simulink model "BaseEngineController_LS"  (Simulink 7.7)
settings: Solver=FixedStepDiscrete  StartTime=0.0  StopTime=10.0  RelTol=1e-3
PreLoadFcn:
  | try, eval([bdroot '_setup']); catch, eval('model_setup', ''); end
InitFcn:
  | try, eval([bdroot '_setup']); catch, eval('model_setup', ''); end
undefined symbols (not defined in the file): ECU555, High, motohawk_build_version, motohawk_trunc_name, motohawk_vardec_config_group, motohawk_vardec_path, True
libraries: MotoHawk_lib x1418, motohawk_control_primitives_lib x183, motohawk_engine_lib x32, simulink x21, motohawk_annotations_lib x9, AutoDoc_lib x8, simulink_extras x4, motohawk_ccp_examples_lib x1, motohawk_control_primitives_motoshare_lib x1
(part 3 of 27)

== system BaseEngineController_LS/Foreground/Inputs/PotentiometerSensors ==
  APP1 : Subsystem  AncestorBlock=motohawk_engine_lib/Non-Linear Sensor Characterization (tbl)  mask(Non-Linear Sensor Characterization (tbl)){nam='APP1', prefix='APP1', units='%', inputunits='ADC', parent_group=motohawk_vardec_path(gcb), tblsize=9, samp_time=-1}
      mask prompts: nam "Name"; units "Output Units"; inputunits "Input Units"; parent_group "MotoTune Group"; tblsize "Table Size"; samp_time "Sample Time"
      mask help:
      | Converts from A/D Counts to Engineering Units using a 1-D Table Lookup.
      | Saturates the converted value around Min and Max values and triggers a Fault when out of range.
      mask init:
      | lbl = ['Non-Linear Sensor (tbl): ' nam ' [' units ']'];
      | group = [parent_group ' | ' nam];
      settings: RTWSystemCode=Function  RTWFcnNameOpts=Use subsystem name  RTWFileNameOpts=Use function name
      mask Display:
      | patch([0 0 1 1], [0 0.075 0.075 0], [230/255 0/255 0/255])
      | patch([0 0 1 1], [0.025 0.05 0.05 0.025], [150/255 0/255 0/255])
      | patch([0 0 1 1], [0 0.025 0.025 0], [0/255 0/255 0/255])
      | 
      | disp(lbl);
  APP1ForcedAdapt : Subsystem
  APP2 : Subsystem  AncestorBlock=motohawk_engine_lib/Non-Linear Sensor Characterization (tbl)  mask(Non-Linear Sensor Characterization (tbl)){nam='APP2', prefix='APP2', units='%', inputunits='ADC', parent_group=motohawk_vardec_path(gcb), tblsize=9, samp_time=-1}
      mask prompts: nam "Name"; units "Output Units"; inputunits "Input Units"; parent_group "MotoTune Group"; tblsize "Table Size"; samp_time "Sample Time"
      mask help:
      | Converts from A/D Counts to Engineering Units using a 1-D Table Lookup.
      | Saturates the converted value around Min and Max values and triggers a Fault when out of range.
      mask init:
      | lbl = ['Non-Linear Sensor (tbl): ' nam ' [' units ']'];
      | group = [parent_group ' | ' nam];
      settings: RTWSystemCode=Function  RTWFcnNameOpts=Use subsystem name  RTWFileNameOpts=Use function name
      mask Display:
      | patch([0 0 1 1], [0 0.075 0.075 0], [230/255 0/255 0/255])
      | patch([0 0 1 1], [0.025 0.05 0.05 0.025], [150/255 0/255 0/255])
      | patch([0 0 1 1], [0 0.025 0.025 0], [0/255 0/255 0/255])
      | 
      | disp(lbl);
  APP2ForcedAdapt : Subsystem
  Bus Creator1 : BusCreator
  Constant4 : Constant  Value=false
  Constant5 : Constant  Value=false
  Linear Sensor Characterization w Adapt : motohawk_engine_lib/Linear Sensor Characterization w Adapt  SystemSampleTime=-1  nam='APP1_Adapt'  prefix='APP1_Adapt'  samp_time=-1  parent_group=motohawk_vardec_path(gcb)
  Linear Sensor Characterization w Adapt1 : motohawk_engine_lib/Linear Sensor Characterization w Adapt  SystemSampleTime=-1  nam='APP2_Adapt'  prefix='APP2_Adapt'  samp_time=-1  parent_group=motohawk_vardec_path(gcb)
  Switch : Switch  Criteria=u2 ~= 0
  Switch1 : Switch  Criteria=u2 ~= 0
  TPS1 : motohawk_engine_lib/Linear Sensor Characterization w Adapt  SystemSampleTime=-1  nam='TPS1'  prefix='TPS1'  samp_time=-1  parent_group=motohawk_vardec_path(gcb)
  TPS2 : motohawk_engine_lib/Linear Sensor Characterization w Adapt  SystemSampleTime=-1  nam='TPS2'  prefix='TPS2'  samp_time=-1  parent_group=motohawk_vardec_path(gcb)
  Terminator{2..5,10..11} (6 alike) : Terminator
  motohawk_ain1 : MotoHawk_lib/Analog I//O Blocks/motohawk_ain  res_name=[]  text_resource=AN5M  code_resource=RES_ECUP  val_resource=-1  target=ECU555-80  resource_enum_str=(None)=-1,ECUP=53,DRVP=54,XDRP=55,AN1M=56,AN2M=57,AN3M=58,AN4M=59,AN5M=60,AN6M=61,AN7M=62,AN8M=63,AN9M=64,AN10M=65,AN11M=66,AN12M=67,AN13M=68,AN14M=69,AN15M=70,AN16M=71,AN17M=72,AN18M=73,AN19M=74,O2A=90,O2B=91,XDRP_B=92  altref=5V Reference  typ=uint16  num_adc_bits=10  use_stat=off  use_vardec=on  nam='APP1AnalogInput'  read_level=1  write_level=1  group='System | I/O Pins | Inputs Config'
  motohawk_ain2 : MotoHawk_lib/Analog I//O Blocks/motohawk_ain  res_name=[]  text_resource=AN4M  code_resource=RES_ECUP  val_resource=-1  target=ECU555-80  resource_enum_str=(None)=-1,ECUP=53,DRVP=54,XDRP=55,AN1M=56,AN2M=57,AN3M=58,AN4M=59,AN5M=60,AN6M=61,AN7M=62,AN8M=63,AN9M=64,AN10M=65,AN11M=66,AN12M=67,AN13M=68,AN14M=69,AN15M=70,AN16M=71,AN17M=72,AN18M=73,AN19M=74,O2A=90,O2B=91,XDRP_B=92  altref=5V Reference  typ=uint16  num_adc_bits=10  use_stat=off  use_vardec=on  nam='APP2AnalogInput'  read_level=1  write_level=1  group='System | I/O Pins | Inputs Config'
  motohawk_ain6 : MotoHawk_lib/Analog I//O Blocks/motohawk_ain  res_name=[]  text_resource=AN5M  code_resource=RES_ECUP  val_resource=-1  target=ECU555-80  resource_enum_str=(None)=-1,ECUP=53,DRVP=54,XDRP=55,AN1M=56,AN2M=57,AN3M=58,AN4M=59,AN5M=60,AN6M=61,AN7M=62,AN8M=63,AN9M=64,AN10M=65,AN11M=66,AN12M=67,AN13M=68,AN14M=69,AN15M=70,AN16M=71,AN17M=72,AN18M=73,AN19M=74,O2A=90,O2B=91,XDRP_B=92  altref=5V Reference  typ=uint16  num_adc_bits=10  use_stat=off  use_vardec=on  nam='TPS1AnalogInput'  read_level=1  write_level=1  group='System | I/O Pins | Inputs Config'
  motohawk_ain9 : MotoHawk_lib/Analog I//O Blocks/motohawk_ain  res_name=[]  text_resource=AN4M  code_resource=RES_ECUP  val_resource=-1  target=ECU555-80  resource_enum_str=(None)=-1,ECUP=53,DRVP=54,XDRP=55,AN1M=56,AN2M=57,AN3M=58,AN4M=59,AN5M=60,AN6M=61,AN7M=62,AN8M=63,AN9M=64,AN10M=65,AN11M=66,AN12M=67,AN13M=68,AN14M=69,AN15M=70,AN16M=71,AN17M=72,AN18M=73,AN19M=74,O2A=90,O2B=91,XDRP_B=92  altref=5V Reference  typ=uint16  num_adc_bits=10  use_stat=off  use_vardec=on  nam='TPS2AnalogInput'  read_level=1  write_level=1  group='System | I/O Pins | Inputs Config'
  motohawk_calibration : MotoHawk_lib/Calibration & Probing Blocks/motohawk_calibration  nam='APP_AdaptMode'  val=0  storage=Calibration  show_more=on  name_source=Use Parameter  data_type=boolean  read_level=1  write_level=1  ovr_cals=on  view_as=Enumeration  enum_struct={'Disabled', 'Enabled'}  vector_style=Wide Row  use_help_units=off  help=''  units=''  use_header_enum=off  row_header_enum={}  col_header_enum={}  use_min_max=off  min_val=-inf  max_val=inf  use_precision=off  precision=''  gain=1  offset=0  exp=1  use_mototune_group=on  mototune_group=motohawk_vardec_path(gcb)
  motohawk_callout1 : motohawk_annotations_lib/motohawk_callout1  BlockType_='Mototron_harea'  desc='\fontsize{12}Read from H/W'  edit_text=Compute the mean forward body acceleration.Worry about rounding.  edit_as=255
  motohawk_callout2 : motohawk_annotations_lib/motohawk_callout1  BlockType_='Mototron_harea'  desc='\fontsize{12}Convert to Engineering Units'  edit_text=Compute the mean forward body acceleration.Worry about rounding.  edit_as=255
  motohawk_callout3 : motohawk_annotations_lib/motohawk_callout1  BlockType_='Mototron_harea'  desc='\fontsize{12}Create a Bus of Sensors'  edit_text=Compute the mean forward body acceleration.Worry about rounding.  edit_as=255
  motohawk_data_read : MotoHawk_lib/Data Storage Blocks/motohawk_data_read  source=Lookup By Name  structure=Scalar  operation=Read scalar from location by index  sz_vec=4  sz_row=2  sz_col=3  typ=boolean  nam='TPSAdaptLoRequest'  checkNull=on  struct_inst_name='Struct1'  struct_nam='MyStruct'
  SensorBus : Outport
  wires:
  Bus Creator1/1 -> SensorBus/1  "PotSensors"
  motohawk_ain1/1 -> APP1/1(ADC), Linear Sensor Characterization w Adapt/1
  motohawk_ain2/1 -> APP2/1(ADC), Linear Sensor Characterization w Adapt1/1
  APP1/2(EngUnitsRaw) -> Terminator2/1
  APP2/2(EngUnitsRaw) -> Terminator3/1
  Linear Sensor Characterization w Adapt/2 -> Terminator4/1
  APP1ForcedAdapt/1(LowSide Request) -> Linear Sensor Characterization w Adapt/2
  APP1ForcedAdapt/2(HiSide Request) -> Linear Sensor Characterization w Adapt/3
  APP2ForcedAdapt/1(LowSide Request) -> Linear Sensor Characterization w Adapt1/2
  APP2ForcedAdapt/2(HiSide Request) -> Linear Sensor Characterization w Adapt1/3
  Linear Sensor Characterization w Adapt1/2 -> Terminator5/1
  Constant4/1 -> TPS1/3
  motohawk_data_read/1 -> TPS2/2, TPS1/2
  TPS2/2 -> Terminator11/1
  TPS1/2 -> Terminator10/1
  motohawk_ain6/1 -> TPS1/1
  motohawk_ain9/1 -> TPS2/1
  APP1/1(EngUnitsFilt) -> Switch/3  "APP1"
  Linear Sensor Characterization w Adapt/1 -> Switch/1
  APP2/1(EngUnitsFilt) -> Switch1/3  "APP2"
  Linear Sensor Characterization w Adapt1/1 -> Switch1/1
  motohawk_calibration/1 -> Switch/2, Switch1/2
  Switch/1 -> Bus Creator1/1  "APP1"
  Switch1/1 -> Bus Creator1/2  "APP2"
  TPS1/1 -> Bus Creator1/3  "TPS1"
  TPS2/1 -> Bus Creator1/4  "TPS2"
  Constant5/1 -> TPS2/3

== system BaseEngineController_LS/Foreground/Outputs/AC Control ==
  AC : Inport
  Discrete Actuator - AC : motohawk_engine_lib/Discrete Actuator Characterization  SystemSampleTime=-1  prefix='AC'  nam='AC'  units='bool'  parent_group=motohawk_vardec_path(gcb)  polarity=High-True
  motohawk_dout : MotoHawk_lib/Digital I//O Blocks/motohawk_dout  resource_name=[]  text_resource=(None)  target=ECU555-80  use_diag=off  use_vardec=on  nam='ACPin'  read_level=1  write_level=1  group='System | I/O Pins | Outputs Config'
  wires:
  Discrete Actuator - AC/1 -> motohawk_dout/1
  AC/1 -> Discrete Actuator - AC/1

== system BaseEngineController_LS/Foreground/Outputs/AEM Infinity Dash ==
  Data : Inport
  Dash Custom 1 : Subsystem
  Dash Message 1 : Subsystem
  Dash Message 2 : Subsystem
  Dash Message 3 : Subsystem
  Dash Message 4 : Subsystem
  Dash Message 5 : Subsystem
  Dash Message 6 : Subsystem
  Dash Message 7 : Subsystem
  Dash Message 8 : Subsystem
  Dash Message Boost : Subsystem
  Dash Message DBW : Subsystem
  wires:
  Data/1 -> Dash Message 1/1(Data), Dash Message 2/1(Data), Dash Message 3/1(Data), Dash Message 4/1(Data), Dash Message 6/1(Data), Dash Message Boost/1(Data), Dash Message DBW/1(Data), Dash Custom 1/1(Data), Dash Message 5/1(Data)

== system BaseEngineController_LS/Foreground/Outputs/Coil Control ==
  SparkEnable : Inport
  SparkStartAngle : Inport  Port=2
  SparkAdvance : Inport  Port=3
  CutSequence : Inport  Port=4
  Trigger : TriggerPort  TriggerType=function-call
  Coil Enable Manager : Subsystem
  Data Type Conversion : DataTypeConversion  SaturateOnIntegerOverflow=on  RndMeth=Zero
  Data Type Conversion1 : DataTypeConversion  SaturateOnIntegerOverflow=on  RndMeth=Zero
  Data Type Conversion2 : DataTypeConversion  SaturateOnIntegerOverflow=on  RndMeth=Zero
  EST Fault Management : Subsystem
  Gain : Gain  Gain=16  SaturateOnIntegerOverflow=on  OutDataTypeStr=Inherit: Same as input  ParamDataTypeStr=Inherit: Same as input
  Gain1 : Gain  Gain=16  SaturateOnIntegerOverflow=on  OutDataTypeStr=Inherit: Same as input  ParamDataTypeStr=Inherit: Same as input
  Gain2 : Gain  Gain=1000  SaturateOnIntegerOverflow=on  OutDataTypeStr=Inherit: Same as input  ParamDataTypeStr=Inherit: Same as input
  Logical Operator1 : Logic  Inputs=3  AllPortsSameDT=off  OutDataTypeStr=boolean
  Spark Sequence : MotoHawk_lib/Advanced Digital I//O/Spark Sequence  text_resource=EST 1  code_resource=RES_EST1  val_resource=-1  target=ECU555-80  resource_enum_str=(None)=-1,EST 1=36,EST 2=37,EST 3=38,EST 4=39,EST 5=40,EST 6=41,EST 7=42,EST 8=43  sequence_type=Standard (Coil per cylinder)  stop_mode=Angle Controlled  update_mode=OS  granularity=Fine  min_duration_mode=Static  min_duration=1.5  use_diag=on  open_threshold=500  use_vardec=on  nam='EST_'  read_level=1  write_level=1  group='System | I/O Pins | Outputs Config'
  motohawk_calibration2 : MotoHawk_lib/Calibration & Probing Blocks/motohawk_calibration  nam='SparkMaxDuration'  val=5  storage=Calibration  show_more=on  name_source=Use Parameter  data_type=Inherit via back propagation  read_level=1  write_level=1  ovr_cals=on  view_as=Number  enum_struct={'Disabled', 'Enabled'}  vector_style=Wide Row  use_help_units=on  help="'Maximum duration for a spark pulse.  Must be a multiple of 5ms'"  units='ms'  use_header_enum=off  row_header_enum={}  col_header_enum={}  use_min_max=off  min_val=-inf  max_val=inf  use_precision=off  precision=''  gain=1  offset=0  exp=1  use_mototune_group=on  mototune_group=motohawk_vardec_path(gcb)
  motohawk_override_rel : MotoHawk_lib/Calibration & Probing Blocks/motohawk_override_rel  SystemSampleTime=-1  parent_name='SparkStartAngle'  show_more=on  name_source=Use Parameter  parent_read_level=1  parent_override_level=1  use_help_units=on  parent_help='Provides a relative offset to input signal'  parent_units='degBTDC'  use_min_max=off  parent_min=-inf  parent_max=inf  use_precision=off  parent_precision=''  parent_gain=1  parent_offset=0  parent_exp=1  use_mototune_group=on  parent_group=motohawk_vardec_path(gcb)
  motohawk_override_rel1 : MotoHawk_lib/Calibration & Probing Blocks/motohawk_override_rel  SystemSampleTime=-1  parent_name='SparkStopAngle'  show_more=on  name_source=Use Parameter  parent_read_level=1  parent_override_level=1  use_help_units=on  parent_help='Provides a relative offset to input signal'  parent_units='degBTDC'  use_min_max=off  parent_min=-inf  parent_max=inf  use_precision=off  parent_precision=''  parent_gain=1  parent_offset=0  parent_exp=1  use_mototune_group=on  parent_group=motohawk_vardec_path(gcb)
  motohawk_probe : MotoHawk_lib/Calibration & Probing Blocks/motohawk_probe  nam='CoilStartAngle'  show_more=on  name_source=Use Parameter  read_level=1  view_as=Number  enum_struct={'Disabled', 'Enabled'}  vector_style=Wide Row  use_help_units=on  help='StartAngle for coils to establish dwell.'  units='degBTDC'  use_header_enum=off  row_header_enum={}  col_header_enum={}  use_precision=off  precision=''  gain=1  offset=0  exp=1  use_mototune_group=on  mototune_group=motohawk_vardec_path(gcb)
  motohawk_probe1 : MotoHawk_lib/Calibration & Probing Blocks/motohawk_probe  nam='CoilStopAngle'  show_more=on  name_source=Use Parameter  read_level=1  view_as=Number  enum_struct={'Disabled', 'Enabled'}  vector_style=Wide Row  use_help_units=on  help='Stop angle for coils to establish dwell.'  units='degBTDC'  use_header_enum=off  row_header_enum={}  col_header_enum={}  use_precision=off  precision=''  gain=1  offset=0  exp=1  use_mototune_group=on  mototune_group=motohawk_vardec_path(gcb)
  motohawk_probe2 : MotoHawk_lib/Calibration & Probing Blocks/motohawk_probe  nam='CoilEnabled'  show_more=on  name_source=Use Parameter  read_level=1  view_as=Number  enum_struct={'Disabled', 'Enabled'}  vector_style=Wide Row  use_help_units=on  help='Enable sate for coils.'  units='bool'  use_header_enum=off  row_header_enum={}  col_header_enum={}  use_precision=off  precision=''  gain=1  offset=0  exp=1  use_mototune_group=on  mototune_group=motohawk_vardec_path(gcb)
  wires:
  CutSequence/1 -> Logical Operator1/3
  SparkEnable/1 -> Logical Operator1/2
  Coil Enable Manager/1(Enable) -> Logical Operator1/1
  Gain2/1 -> Data Type Conversion2/1
  Data Type Conversion2/1 -> Spark Sequence/4
  motohawk_override_rel/1 -> motohawk_probe/1, Gain/1
  motohawk_override_rel1/1 -> motohawk_probe1/1, Gain1/1
  Logical Operator1/1 -> motohawk_probe2/1, Spark Sequence/1
  SparkAdvance/1 -> motohawk_override_rel1/1
  SparkStartAngle/1 -> motohawk_override_rel/1
  motohawk_calibration2/1 -> Gain2/1
  Data Type Conversion1/1 -> Spark Sequence/3
  Data Type Conversion/1 -> Spark Sequence/2
  Gain1/1 -> Data Type Conversion1/1
  Gain/1 -> Data Type Conversion/1
  Spark Sequence/1 -> EST Fault Management/1(Short)
  Spark Sequence/2 -> EST Fault Management/2(Open)
  Spark Sequence/3 -> EST Fault Management/3(OpenADC)
  Spark Sequence/4 -> EST Fault Management/4(Dwell)

== system BaseEngineController_LS/Foreground/Outputs/ETC_CutPower ==
  ETC : Inport
  ESTOP : Inport  Port=2
  TimeSinceStall : Inport  Port=3
  Logical Operator : Logic  AllPortsSameDT=off  OutDataTypeStr=boolean
  Logical Operator9 : Logic  Operator=OR  AllPortsSameDT=off  OutDataTypeStr=boolean
  Relational Operator : RelationalOperator  Operator=<  OutDataTypeStr=boolean
  Relational Operator3 : RelationalOperator  Operator=>  ZeroCross=off  InputSameDT=on
  motohawk_calibration1 : MotoHawk_lib/Calibration & Probing Blocks/motohawk_calibration  nam='ETC_CutPower_ETC'  val=20  storage=Calibration  show_more=on  name_source=Use Parameter  data_type=Inherit from 'Default Value'  read_level=1  write_level=1  ovr_cals=on  view_as=Number  enum_struct={'Disabled', 'Enabled'}  vector_style=Wide Row  use_help_units=on  help='Cut power to ETC if ETC request is less than this'  units='%'  use_header_enum=off  row_header_enum={}  col_header_enum={}  use_min_max=on  min_val=0  max_val=100  use_precision=on  precision='2.3'  gain=1  offset=0  exp=1  use_mototune_group=on  mototune_group=motohawk_vardec_path(gcb)
  motohawk_calibration3 : MotoHawk_lib/Calibration & Probing Blocks/motohawk_calibration  nam='ETC_CutPower_StallTime'  val=15  storage=Calibration  show_more=on  name_source=Use Parameter  data_type=Inherit from 'Default Value'  read_level=1  write_level=1  ovr_cals=on  view_as=Number  enum_struct={'Disabled', 'Enabled'}  vector_style=Wide Row  use_help_units=on  help='Cut power to ETC after stalled this long'  units='s'  use_header_enum=off  row_header_enum={}  col_header_enum={}  use_min_max=off  min_val=0  max_val=100  use_precision=on  precision='2.3'  gain=1  offset=0  exp=1  use_mototune_group=on  mototune_group=motohawk_vardec_path(gcb)
  ETC OFF : Outport
  wires:
  ESTOP/1 -> Logical Operator9/1
  TimeSinceStall/1 -> Relational Operator3/1
  motohawk_calibration3/1 -> Relational Operator3/2
  Logical Operator9/1 -> ETC OFF/1
  Relational Operator3/1 -> Logical Operator/1
  ETC/1 -> Relational Operator/1
  motohawk_calibration1/1 -> Relational Operator/2
  Relational Operator/1 -> Logical Operator/2
  Logical Operator/1 -> Logical Operator9/2

== system BaseEngineController_LS/Foreground/Outputs/FAN Control ==
  FAN-1 : Inport
  FAN-2 : Inport  Port=2
  IAC-P-CONTROL : motohawk_engine_lib/PWM Characterization  SystemSampleTime=-1  nam='FAN1_PWM'  prefix='FAN1_PWM'  units='%'  parent_group=motohawk_vardec_path(gcb)
  IAC-P-CONTROL1 : motohawk_engine_lib/PWM Characterization  SystemSampleTime=-1  nam='FAN2_PWM'  prefix='FAN2_PWM'  units='%'  parent_group=motohawk_vardec_path(gcb)
  motohawk_pwm : MotoHawk_lib/Analog I//O Blocks/motohawk_pwm  res_name=[]  text_resource=(None)  code_resource=NONE  val_resource=-1  target=ECU555-80  resource_enum_str=(None)=-1,FUELP=0,ETC=1,HSOL1=2,HSOL2=3,HSOL3=4,HSOL4=5,START=6,OILP=11,FINJ1=12,FINJ2=13,FINJ3=14,FINJ4=15,FINJ5=16,FINJ6=17,AINJ1=18,AINJ2=19,AINJ3=20,AINJ4=21,AINJ5=22,AINJ6=23,TACH=24,EST 1=36,EST 2=37,EST 3=38,EST 4=39,EST 5=40,EST 6=41,EST 7=42,EST 8=43  freq_mode=-1  min_freq=2  use_max_freq=off  max_freq=42949672.96  use_enable=off  use_brake=off  output_current=off  output_fault_status=off  use_child=off  use_vardec=on  nam='FAN1Pin_PWM'  read_level=1  write_level=1  group='System | I/O Pins | Outputs Config'
  motohawk_pwm1 : MotoHawk_lib/Analog I//O Blocks/motohawk_pwm  res_name=[]  text_resource=(None)  code_resource=NONE  val_resource=-1  target=ECU555-80  resource_enum_str=(None)=-1,FUELP=0,ETC=1,HSOL1=2,HSOL2=3,HSOL3=4,HSOL4=5,START=6,OILP=11,FINJ1=12,FINJ2=13,FINJ3=14,FINJ4=15,FINJ5=16,FINJ6=17,AINJ1=18,AINJ2=19,AINJ3=20,AINJ4=21,AINJ5=22,AINJ6=23,TACH=24,EST 1=36,EST 2=37,EST 3=38,EST 4=39,EST 5=40,EST 6=41,EST 7=42,EST 8=43  freq_mode=-1  min_freq=2  use_max_freq=off  max_freq=42949672.96  use_enable=off  use_brake=off  output_current=off  output_fault_status=off  use_child=off  use_vardec=on  nam='FAN2Pin_PWM'  read_level=1  write_level=1  group='System | I/O Pins | Outputs Config'
  wires:
  FAN-1/1 -> IAC-P-CONTROL/1
  FAN-2/1 -> IAC-P-CONTROL1/1
  IAC-P-CONTROL/1 -> motohawk_pwm/1
  IAC-P-CONTROL/2 -> motohawk_pwm/2
  IAC-P-CONTROL1/1 -> motohawk_pwm1/1
  IAC-P-CONTROL1/2 -> motohawk_pwm1/2

== system BaseEngineController_LS/Foreground/Outputs/FuelPump ==
  State : Inport
  Discrete Actuator - FUELP : motohawk_engine_lib/Discrete Actuator Characterization  SystemSampleTime=-1  prefix='FUELP'  nam='FUELP'  units='bool'  parent_group=motohawk_vardec_path(gcb)  polarity=High-True
  motohawk_dout : MotoHawk_lib/Digital I//O Blocks/motohawk_dout  resource_name=[]  text_resource=(None)  target=ECU555-80  use_diag=off  use_vardec=on  nam='FuelPumpPin'  read_level=1  write_level=1  group='System | I/O Pins | Outputs Config'
  wires:
  State/1 -> Discrete Actuator - FUELP/1
  Discrete Actuator - FUELP/1 -> motohawk_dout/1

== system BaseEngineController_LS/Foreground/Outputs/HBridge ==
  ETCDuty Cycle : Inport
  SysVoltIdx : Inport  Port=2
  ETC_CutPower : Inport  Port=3
  Abs : Abs
  Abs1 : Abs
  Constant : Constant  Value=5
  Constant2 : Constant  Value=0  SampleTime=-1
  Convert to integer 0.01Hz resolution : Gain  Gain=100  SaturateOnIntegerOverflow=on  OutDataTypeStr=Inherit: Same as input  ParamDataTypeStr=Inherit: Same as input
  Convert to integer 14-bit PWM resolution : Gain  Gain=40.95  SaturateOnIntegerOverflow=on  OutDataTypeStr=Inherit: Same as input  ParamDataTypeStr=Inherit: Same as input
  Data Type Conversion3 : DataTypeConversion  OutDataTypeStr=uint32  SaturateOnIntegerOverflow=on  RndMeth=Zero
  Data Type Conversion4 : DataTypeConversion  OutDataTypeStr=int16  SaturateOnIntegerOverflow=on  RndMeth=Zero
  Logical Operator : Logic  Operator=NOT  AllPortsSameDT=off  OutDataTypeStr=boolean
  Logical Operator1 : Logic  AllPortsSameDT=off  OutDataTypeStr=boolean
  Logical Operator4 : Logic  Inputs=3  AllPortsSameDT=off  OutDataTypeStr=boolean
  Product : Product  SaturateOnIntegerOverflow=on  InputSameDT=on  OutDataTypeStr=Inherit: Same as first input
  Relational Operator3 : RelationalOperator  Operator=>  OutDataTypeStr=boolean
  Relational Operator4 : RelationalOperator  Operator=<  OutDataTypeStr=boolean
  Relational Operator5 : RelationalOperator  Operator=>  OutDataTypeStr=boolean
  Saturation : Saturate  UpperLimit=100  LowerLimit=-100
  Sum : Sum  Inputs=|++  SaturateOnIntegerOverflow=on
  Switch : Switch  Threshold=1
  Time Since Enabled (With Input)1 : motohawk_control_primitives_lib/Time Since Enabled (With Input)1  SystemSampleTime=-1  nam='ETCOpenFaultTimer'  samp_time=-1  init=0  upperlim=16000
  motohawk_calibration1 : MotoHawk_lib/Calibration & Probing Blocks/motohawk_calibration  nam='ETC_I_MIN'  val=5  storage=Calibration  show_more=on  name_source=Use Parameter  data_type=double  read_level=1  write_level=1  ovr_cals=on  view_as=Number  enum_struct={'Disabled', 'Enabled'}  vector_style=Wide Row  use_help_units=on  help="'H-bridge open circuit fault:  ETC current must exceed this when ETC duty cycle is > ETC_OC_MIN, otherwise an open circuit fault may exist.'"  units='mA'  use_header_enum=off  row_header_enum={}  col_header_enum={}  use_min_max=off  min_val=0  max_val=inf  use_precision=off  precision=''  gain=1  offset=0  exp=1  use_mototune_group=on  mototune_group=motohawk_vardec_path(gcb)
  motohawk_calibration2 : MotoHawk_lib/Calibration & Probing Blocks/motohawk_calibration  nam='ETC_Offset'  val=0  storage=Calibration  show_more=on  name_source=Use Parameter  data_type=double  read_level=1  write_level=1  ovr_cals=on  view_as=Number  enum_struct={'Disabled', 'Enabled'}  vector_style=Wide Row  use_help_units=on  help='Offset from engineering units to PWM duty cycle'  units='%'  use_header_enum=off  row_header_enum={}  col_header_enum={}  use_min_max=off  min_val=-inf  max_val=inf  use_precision=off  precision=''  gain=1  offset=0  exp=1  use_mototune_group=on  mototune_group=motohawk_vardec_path(gcb)
  motohawk_calibration3 : MotoHawk_lib/Calibration & Probing Blocks/motohawk_calibration  nam='ETC_OC_MIN'  val=50  storage=Calibration  show_more=on  name_source=Use Parameter  data_type=double  read_level=1  write_level=1  ovr_cals=on  view_as=Number  enum_struct={'Disabled', 'Enabled'}  vector_style=Wide Row  use_help_units=on  help="'H-bridge open circuit fault:  ETC duty cycle must exceed this to enable open circuit fault detection.'"  units='%'  use_header_enum=off  row_header_enum={}  col_header_enum={}  use_min_max=off  min_val=0  max_val=inf  use_precision=off  precision=''  gain=1  offset=0  exp=1  use_mototune_group=on  mototune_group=motohawk_vardec_path(gcb)
  motohawk_calibration4 : MotoHawk_lib/Calibration & Probing Blocks/motohawk_calibration  nam='ETC_Frequency'  val=2500  storage=Calibration  show_more=on  name_source=Use Parameter  data_type=double  read_level=1  write_level=1  ovr_cals=on  view_as=Number  enum_struct={'Disabled', 'Enabled'}  vector_style=Wide Row  use_help_units=on  help='Frequency of PWM output'  units='Hz'  use_header_enum=off  row_header_enum={}  col_header_enum={}  use_min_max=on  min_val=7.63  max_val=inf  use_precision=off  precision=''  gain=1  offset=0  exp=1  use_mototune_group=on  mototune_group=motohawk_vardec_path(gcb)
  motohawk_calibration5 : MotoHawk_lib/Calibration & Probing Blocks/motohawk_calibration  nam='ETC_CutPower_Permitted'  val=1  storage=Calibration  show_more=on  name_source=Use Parameter  data_type=boolean  read_level=1  write_level=1  ovr_cals=on  view_as=Number  enum_struct={'Disabled', 'Enabled'}  vector_style=Wide Row  use_help_units=on  help='Cut power to ETC after ESTOP or long stalled period'  units='flag'  use_header_enum=off  row_header_enum={}  col_header_enum={}  use_min_max=off  min_val=0  max_val=100  use_precision=on  precision='2.3'  gain=1  offset=0  exp=1  use_mototune_group=on  mototune_group=motohawk_vardec_path(gcb)
  motohawk_fault_def1 : MotoHawk_lib/Fault Management Blocks/motohawk_fault_def  nam='ETC_Open_Fault'  mode=Enabled  id=[]  x=25  y=50  input_suspected=on  indeterminate=off  increment_xy=on  downsample_count=1  ovr_cals=on  ovr_actions=on  show_actions=off  action1_name=''  action1_cond=(None)  action2_name=''  action2_cond=(None)  action3_name=''  action3_cond=(None)  action4_name=''  action4_cond=(None)
  motohawk_interpolation_1d : MotoHawk_lib/Lookup Tables/motohawk_interpolation_1d  nam='ETC_VoltageComp'  table_data=ones(1,9)  show_more=on  data_type=Inherit from 'Table Data'  storage=NonAdaptive  read_level=1  write_level=1  ovr_cals=on  use_help=on  help='Gain on ETC duty cycle based on DRVP'  units=''  use_min_max=off  min_val=-inf  max_val=inf  use_precision=off  precision=''  gain=1  offset=0  exp=1  use_links=off  prelookup_block=''  output_name=''  use_mototune_group=on  mototune_group=motohawk_vardec_path(gcb)
  motohawk_override_abs2 : MotoHawk_lib/Calibration & Probing Blocks/motohawk_override_abs  SystemSampleTime=-1  parent_name='ETC'  parent_val=0  show_more=on  name_source=Use Parameter  parent_read_level=1  parent_override_level=1  view_as=Number  enum_struct={'Disabled', 'Enabled'}  use_help_units=on  parent_help='Override result of linear sensor characterization, in engineering units'  parent_units=''  use_min_max=on  parent_min=-inf  parent_max=inf  use_precision=off  parent_precision=''  parent_gain=1  parent_offset=0  parent_exp=1  use_mototune_group=on  parent_group=motohawk_vardec_path(gcb)
  motohawk_probe : MotoHawk_lib/Calibration & Probing Blocks/motohawk_probe  nam='ETB_Curr_Flt'  show_more=off  name_source=Use Parameter  read_level=1  view_as=Number  enum_struct={'Disabled', 'Enabled'}  vector_style=Wide Row  use_help_units=off  help=''  units=''  use_header_enum=off  row_header_enum={}  col_header_enum={}  use_precision=off  precision=''  gain=1  offset=0  exp=1  use_mototune_group=off  mototune_group=motohawk_vardec_path(gcb)
  motohawk_probe1 : MotoHawk_lib/Calibration & Probing Blocks/motohawk_probe  nam='ETC_Current'  show_more=on  name_source=Use Parameter  read_level=1  view_as=Number  enum_struct={'Disabled', 'Enabled'}  vector_style=Wide Row  use_help_units=on  help='Current output of ETC duty cycle.'  units='mA'  use_header_enum=off  row_header_enum={}  col_header_enum={}  use_precision=off  precision=''  gain=1  offset=0  exp=1  use_mototune_group=on  mototune_group=motohawk_vardec_path(gcb)
  motohawk_probe2 : MotoHawk_lib/Calibration & Probing Blocks/motohawk_probe  nam='ETC_DutyCycle'  show_more=on  name_source=Use Parameter  read_level=1  view_as=Number  enum_struct={'Disabled', 'Enabled'}  vector_style=Wide Row  use_help_units=on  help='Actual duty cycle of actuator'  units='%'  use_header_enum=off  row_header_enum={}  col_header_enum={}  use_precision=off  precision=''  gain=1  offset=0  exp=1  use_mototune_group=on  mototune_group=motohawk_vardec_path(gcb)
  motohawk_pwm1 : MotoHawk_lib/Analog I//O Blocks/motohawk_pwm  res_name=[]  text_resource=(None)  code_resource=RES_H1  val_resource=1  target=ECU555-80  resource_enum_str=(None)=-1,FUELP=0,ETC=1,HSOL1=2,HSOL2=3,HSOL3=4,HSOL4=5,START=6,OILP=11,FINJ1=12,FINJ2=13,FINJ3=14,FINJ4=15,FINJ5=16,FINJ6=17,AINJ1=18,AINJ2=19,AINJ3=20,AINJ4=21,AINJ5=22,AINJ6=23,TACH=24,EST 1=36,EST 2=37,EST 3=38,EST 4=39,EST 5=40,EST 6=41,EST 7=42,EST 8=43  freq_mode=-1  min_freq=64  use_max_freq=off  max_freq=42949672.96  use_enable=off  use_brake=off  output_current=on  output_fault_status=off  use_child=off  use_vardec=on  nam='ETCPin'  read_level=1  write_level=1  group='System | I/O Pins | Outputs Config'
  wires:
  Abs1/1 -> Relational Operator4/1
  Abs/1 -> Relational Operator3/1
  motohawk_pwm1/1 -> Abs1/1, motohawk_probe1/1
  motohawk_calibration1/1 -> Relational Operator4/2
  motohawk_calibration3/1 -> Relational Operator3/2
  Relational Operator3/1 -> Logical Operator4/2
  Relational Operator4/1 -> Logical Operator4/3, motohawk_probe/1
  Logical Operator4/1 -> Time Since Enabled (With Input)1/1
  Time Since Enabled (With Input)1/1 -> Relational Operator5/1
  Constant/1 -> Relational Operator5/2
  Relational Operator5/1 -> motohawk_fault_def1/1
  SysVoltIdx/1 -> motohawk_interpolation_1d/1
  ETCDuty Cycle/1 -> motohawk_override_abs2/1
  motohawk_interpolation_1d/1 -> Product/2
  Saturation/1 -> Abs/1, motohawk_probe2/1, Convert to integer 14-bit PWM resolution/1  "<ETC>"
  motohawk_calibration4/1 -> Convert to integer 0.01Hz resolution/1
  Data Type Conversion3/1 -> motohawk_pwm1/2
  Convert to integer 0.01Hz resolution/1 -> Data Type Conversion3/1
  motohawk_override_abs2/1 -> Product/1
  Product/1 -> Sum/1
  motohawk_calibration2/1 -> Sum/2
  Data Type Conversion4/1 -> motohawk_pwm1/1
  Convert to integer 14-bit PWM resolution/1 -> Data Type Conversion4/1
  Constant2/1 -> Switch/1
  Sum/1 -> Switch/3
  Switch/1 -> Saturation/1
  Logical Operator/1 -> Logical Operator4/1
  Logical Operator1/1 -> Switch/2, Logical Operator/1
  ETC_CutPower/1 -> Logical Operator1/2
  motohawk_calibration5/1 -> Logical Operator1/1

== system BaseEngineController_LS/Foreground/Outputs/IAC-Control ==
  IAC-P : Inport
  IAC-S : Inport  Port=2
  IAC-P-CONTROL : motohawk_engine_lib/PWM Characterization  SystemSampleTime=-1  nam='IAC_P'  prefix='IAC_P'  units='%'  parent_group=motohawk_vardec_path(gcb)
  IAC-S-CONTROL : motohawk_engine_lib/PWM Characterization  SystemSampleTime=-1  nam='IAC_S'  prefix='IAC_S'  units='%'  parent_group=motohawk_vardec_path(gcb)
  motohawk_pwm : MotoHawk_lib/Analog I//O Blocks/motohawk_pwm  res_name=[]  text_resource=(None)  code_resource=NONE  val_resource=-1  target=ECU555-80  resource_enum_str=(None)=-1,FUELP=0,ETC=1,HSOL1=2,HSOL2=3,HSOL3=4,HSOL4=5,START=6,OILP=11,FINJ1=12,FINJ2=13,FINJ3=14,FINJ4=15,FINJ5=16,FINJ6=17,AINJ1=18,AINJ2=19,AINJ3=20,AINJ4=21,AINJ5=22,AINJ6=23,TACH=24,EST 1=36,EST 2=37,EST 3=38,EST 4=39,EST 5=40,EST 6=41,EST 7=42,EST 8=43  freq_mode=-1  min_freq=2  use_max_freq=off  max_freq=42949672.96  use_enable=off  use_brake=off  output_current=off  output_fault_status=off  use_child=off  use_vardec=on  nam='IAC_PPin'  read_level=1  write_level=1  group='System | I/O Pins | Outputs Config'
  motohawk_pwm1 : MotoHawk_lib/Analog I//O Blocks/motohawk_pwm  res_name=[]  text_resource=(None)  code_resource=NONE  val_resource=-1  target=ECU555-80  resource_enum_str=(None)=-1,FUELP=0,ETC=1,HSOL1=2,HSOL2=3,HSOL3=4,HSOL4=5,START=6,OILP=11,FINJ1=12,FINJ2=13,FINJ3=14,FINJ4=15,FINJ5=16,FINJ6=17,AINJ1=18,AINJ2=19,AINJ3=20,AINJ4=21,AINJ5=22,AINJ6=23,TACH=24,EST 1=36,EST 2=37,EST 3=38,EST 4=39,EST 5=40,EST 6=41,EST 7=42,EST 8=43  freq_mode=-1  min_freq=2  use_max_freq=off  max_freq=42949672.96  use_enable=off  use_brake=off  output_current=off  output_fault_status=off  use_child=off  use_vardec=on  nam='IAC_SPin'  read_level=1  write_level=1  group='System | I/O Pins | Outputs Config'
  wires:
  IAC-S/1 -> IAC-S-CONTROL/1
  IAC-P/1 -> IAC-P-CONTROL/1
  IAC-P-CONTROL/1 -> motohawk_pwm/1
  IAC-P-CONTROL/2 -> motohawk_pwm/2
  IAC-S-CONTROL/1 -> motohawk_pwm1/1
  IAC-S-CONTROL/2 -> motohawk_pwm1/2

== system BaseEngineController_LS/Foreground/Outputs/Injector Control ==
  SOI : Inport
  InjMPW : Inport  Port=2
  InjEPWOffset : Inport  Port=3
  CutSequence : Inport  Port=4
  MakeUpEOI : Inport  Port=5
  Constant : Constant  Value=0
  Data Type Conversion{1..9} (9 alike) : DataTypeConversion  SaturateOnIntegerOverflow=on  RndMeth=Zero
  Gain{1,3..5,7..8} (6 alike) : Gain  Gain=1000  SaturateOnIntegerOverflow=on  OutDataTypeStr=Inherit: Same as input  ParamDataTypeStr=Inherit: Same as input
  Gain2 : Gain  Gain=16  SaturateOnIntegerOverflow=on  OutDataTypeStr=Inherit: Same as input  ParamDataTypeStr=Inherit: Same as input
  Gain6 : Gain  Gain=16  SaturateOnIntegerOverflow=on  OutDataTypeStr=Inherit: Same as input  ParamDataTypeStr=Inherit: Same as input
  Injector Diagnostics : Subsystem  AncestorBlock=MotoHawk_lib/Extra Development Blocks/Injector Diagnostics  mask(Injector Sequence Diagnostics){prefix='Inj', group=motohawk_vardec_path(gcb)}
      mask prompts: group "MotoTune Group"
      mask help:
      | Monitors the output of the Injector Sequence block, and checks for open/short conditions.
      |
      | It outputs vectors for the Open and Short status, appropriate for demuxing and connecting to Fault Definition blocks.
      mask init:
      | lbl = ['Injector\nDiagnostics\n(' prefix ')'];
      mask Display:
      | patch([0 0 1 1], 0.6*[0 0.075 0.075 0], [230/255 0/255 0/255])
      | patch([0 0 1 1], 0.6*[0.025 0.05 0.05 0.025], [150/255 0/255 0/255])
      | patch([0 0 1 1], 0.6*[0 0.025 0.025 0], [0/255 0/255 0/255])
      | 
      | disp(lbl);
  Injector Enable Manager : Subsystem  TreatAsAtomicUnit=on
  Injector Sequence : MotoHawk_lib/Advanced Digital I//O/Injector Sequence  text_resource=FINJ1  code_resource=NONE  val_resource=-1  target=ECU555-80  resource_enum_str=(None)=-1,FINJ1=12,FINJ2=13,FINJ3=14,FINJ4=15,FINJ5=16,FINJ6=17,AINJ1=18,AINJ2=19,AINJ3=20,AINJ4=21,AINJ5=22,AINJ6=23  sequence_type=Standard (Injector per cylinder)  behavior=Standard  update_mode=OS  granularity=Fine  use_makeup=off  min_eoi_soi_angle=400  use_diag=on  show_trans_enable=off  min_duration_mode=Dynamic  min_duration=1.5  use_vardec=on  nam='INJ_'  read_level=1  write_level=1  group='System | I/O Pins | Outputs Config'
  Logical Operator : Logic  Inputs=3  AllPortsSameDT=off  OutDataTypeStr=boolean
  Logical Operator1 : Logic  Operator=NOT  AllPortsSameDT=off  OutDataTypeStr=boolean
  Terminator : Terminator
  motohawk_calibration1 : MotoHawk_lib/Calibration & Probing Blocks/motohawk_calibration  nam='InjectiorMinDuration'  val=1  storage=Calibration  show_more=on  name_source=Use Parameter  data_type=Inherit from 'Default Value'  read_level=1  write_level=1  ovr_cals=on  view_as=Number  enum_struct={'Disabled', 'Enabled'}  vector_style=Wide Row  use_help_units=on  help='Fuel injector min pulsewidth'  units='ms'  use_header_enum=off  row_header_enum={}  col_header_enum={}  use_min_max=off  min_val=-inf  max_val=inf  use_precision=off  precision=''  gain=1  offset=0  exp=1  use_mototune_group=on  mototune_group=motohawk_vardec_path(gcb)
  motohawk_calibration6 : MotoHawk_lib/Calibration & Probing Blocks/motohawk_calibration  nam='MinMakeUpPW'  val=0.1  storage=Calibration  show_more=on  name_source=Use Parameter  data_type=Inherit from 'Default Value'  read_level=1  write_level=1  ovr_cals=on  view_as=Number  enum_struct={'Disabled', 'Enabled'}  vector_style=Wide Row  use_help_units=on  help='Minimum change in injector pulse width that will trigger a make-up pulse.'  units='ms'  use_header_enum=off  row_header_enum={}  col_header_enum={}  use_min_max=off  min_val=-inf  max_val=inf  use_precision=off  precision=''  gain=1  offset=0  exp=1  use_mototune_group=on  mototune_group=motohawk_vardec_path(gcb)
  motohawk_calibration9 : MotoHawk_lib/Calibration & Probing Blocks/motohawk_calibration  nam='InjectorMaxDuration'  val=50  storage=Calibration  show_more=on  name_source=Use Parameter  data_type=Inherit from 'Default Value'  read_level=1  write_level=1  ovr_cals=on  view_as=Number  enum_struct={'Disabled', 'Enabled'}  vector_style=Wide Row  use_help_units=on  help="'Maximum duration for an injector pulse.  Must be a multiple of 5ms'"  units='ms'  use_header_enum=off  row_header_enum={}  col_header_enum={}  use_min_max=off  min_val=-inf  max_val=inf  use_precision=off  precision=''  gain=1  offset=0  exp=1  use_mototune_group=on  mototune_group=motohawk_vardec_path(gcb)
  motohawk_data_read : MotoHawk_lib/Data Storage Blocks/motohawk_data_read  source=Lookup By Name  structure=Scalar  operation=Read scalar from location by index  sz_vec=4  sz_row=2  sz_col=3  typ=boolean  nam='ESTOP'  checkNull=on  struct_inst_name='MyData'  struct_nam='MyStruct'
  motohawk_override_abs1 : MotoHawk_lib/Calibration & Probing Blocks/motohawk_override_abs  SystemSampleTime=-1  parent_name='Elec_PW'  parent_val=0  show_more=on  name_source=Use Parameter  parent_read_level=1  parent_override_level=1  view_as=Number  enum_struct={'Disabled', 'Enabled'}  use_help_units=off  parent_help=''  parent_units=''  use_min_max=off  parent_min=-inf  parent_max=inf  use_precision=off  parent_precision=''  parent_gain=1  parent_offset=0  parent_exp=1  use_mototune_group=on  parent_group=motohawk_vardec_path(gcb)
  motohawk_override_abs2 : MotoHawk_lib/Calibration & Probing Blocks/motohawk_override_abs  SystemSampleTime=-1  parent_name='MakeUp_EOI'  parent_val=0  show_more=on  name_source=Use Parameter  parent_read_level=1  parent_override_level=1  view_as=Number  enum_struct={'Disabled', 'Enabled'}  use_help_units=off  parent_help=''  parent_units=''  use_min_max=off  parent_min=-inf  parent_max=inf  use_precision=off  parent_precision=''  parent_gain=1  parent_offset=0  parent_exp=1  use_mototune_group=on  parent_group=motohawk_vardec_path(gcb)
  motohawk_override_abs3 : MotoHawk_lib/Calibration & Probing Blocks/motohawk_override_abs  SystemSampleTime=-1  parent_name='SOI'  parent_val=0  show_more=on  name_source=Use Parameter  parent_read_level=1  parent_override_level=1  view_as=Number  enum_struct={'Disabled', 'Enabled'}  use_help_units=off  parent_help=''  parent_units=''  use_min_max=off  parent_min=-inf  parent_max=inf  use_precision=off  parent_precision=''  parent_gain=1  parent_offset=0  parent_exp=1  use_mototune_group=on  parent_group=motohawk_vardec_path(gcb)
  motohawk_override_abs4 : MotoHawk_lib/Calibration & Probing Blocks/motohawk_override_abs  SystemSampleTime=-1  parent_name='Mech_PW'  parent_val=0  show_more=on  name_source=Use Parameter  parent_read_level=1  parent_override_level=1  view_as=Number  enum_struct={'Disabled', 'Enabled'}  use_help_units=off  parent_help=''  parent_units=''  use_min_max=off  parent_min=-inf  parent_max=inf  use_precision=off  parent_precision=''  parent_gain=1  parent_offset=0  parent_exp=1  use_mototune_group=on  parent_group=motohawk_vardec_path(gcb)
  motohawk_override_abs5 : MotoHawk_lib/Calibration & Probing Blocks/motohawk_override_abs  SystemSampleTime=-1  parent_name='InjEnable'  parent_val=0  show_more=on  name_source=Use Parameter  parent_read_level=1  parent_override_level=1  view_as=Number  enum_struct={'Disabled', 'Enabled'}  use_help_units=off  parent_help=''  parent_units=''  use_min_max=off  parent_min=-inf  parent_max=inf  use_precision=off  parent_precision=''  parent_gain=1  parent_offset=0  parent_exp=1  use_mototune_group=on  parent_group=motohawk_vardec_path(gcb)
  motohawk_override_abs6 : MotoHawk_lib/Calibration & Probing Blocks/motohawk_override_abs  SystemSampleTime=-1  parent_name='ESTOP_FuelInj_Ovr'  parent_val=0  show_more=on  name_source=Use Parameter  parent_read_level=1  parent_override_level=1  view_as=Number  enum_struct={'Disabled', 'Enabled'}  use_help_units=off  parent_help=''  parent_units=''  use_min_max=off  parent_min=-inf  parent_max=inf  use_precision=off  parent_precision=''  parent_gain=1  parent_offset=0  parent_exp=1  use_mototune_group=on  parent_group=motohawk_vardec_path(gcb)
  motohawk_probe2 : MotoHawk_lib/Calibration & Probing Blocks/motohawk_probe  nam='InjectorsEnabled'  show_more=on  name_source=Use Parameter  read_level=1  view_as=Number  enum_struct={'Disabled', 'Enabled'}  vector_style=Wide Row  use_help_units=on  help='Enable state for injectors.'  units='bool'  use_header_enum=off  row_header_enum={}  col_header_enum={}  use_precision=off  precision=''  gain=1  offset=0  exp=1  use_mototune_group=on  mototune_group=motohawk_vardec_path(gcb)
  wires:
  motohawk_override_abs4/1 -> Gain3/1
  motohawk_override_abs3/1 -> Gain2/1
  motohawk_override_abs2/1 -> Gain6/1
  motohawk_override_abs1/1 -> Gain1/1
  Data Type Conversion8/1 -> Injector Sequence/8
  Gain7/1 -> Data Type Conversion8/1
  Data Type Conversion7/1 -> Injector Sequence/7
  Gain6/1 -> Data Type Conversion7/1
  Data Type Conversion6/1 -> Injector Sequence/5
  Gain5/1 -> Data Type Conversion6/1
  Data Type Conversion5/1 -> Injector Sequence/4
  Gain4/1 -> Data Type Conversion5/1
  Injector Sequence/2 -> Terminator/1
  Injector Sequence/1 -> Injector Diagnostics/2(TX Count)
  Gain1/1 -> Data Type Conversion1/1
  Data Type Conversion1/1 -> Injector Sequence/6
  motohawk_calibration9/1 -> Gain5/1
  Data Type Conversion4/1 -> Injector Diagnostics/1(Inj_Enabled), motohawk_probe2/1, Injector Sequence/1
  motohawk_calibration6/1 -> Gain7/1
  MakeUpEOI/1 -> motohawk_override_abs2/1
  Logical Operator/1 -> motohawk_override_abs5/1
  InjEPWOffset/1 -> motohawk_override_abs1/1
  InjMPW/1 -> motohawk_override_abs4/1
  SOI/1 -> motohawk_override_abs3/1
  Constant/1 -> Gain4/1
  Data Type Conversion3/1 -> Injector Sequence/3
  Data Type Conversion2/1 -> Injector Sequence/2
  Gain2/1 -> Data Type Conversion2/1
  Gain3/1 -> Data Type Conversion3/1
  motohawk_override_abs5/1 -> Data Type Conversion4/1
  Injector Enable Manager/1(Enable) -> Logical Operator/3
  CutSequence/1 -> Logical Operator/2
  motohawk_data_read/1 -> Logical Operator1/1
  Logical Operator1/1 -> motohawk_override_abs6/1
  motohawk_override_abs6/1 -> Logical Operator/1
  motohawk_calibration1/1 -> Gain8/1
  Gain8/1 -> Data Type Conversion9/1
  Data Type Conversion9/1 -> Injector Sequence/9

== system BaseEngineController_LS/Foreground/Outputs/WASTEGATE-Control ==
  WASTEGATE : Inport
  Logical Operator : Logic  Operator=NOT  AllPortsSameDT=off  OutDataTypeStr=boolean
  PWM Characterization : motohawk_engine_lib/PWM Characterization  SystemSampleTime=-1  nam='WASTEGATE'  prefix='WASTEGATE'  units='%'  parent_group=motohawk_vardec_path(gcb)
  Product : Product  RndMeth=Zero
  motohawk_fault_action : MotoHawk_lib/Fault Management Blocks/motohawk_fault_action  nam='DisableWastegate'  output_status=on  eval_nam=DisableWastegate
  motohawk_pwm : MotoHawk_lib/Analog I//O Blocks/motohawk_pwm  res_name=[]  text_resource=(None)  code_resource=NONE  val_resource=-1  target=ECU555-80  resource_enum_str=(None)=-1,FUELP=0,ETC=1,HSOL1=2,HSOL2=3,HSOL3=4,HSOL4=5,START=6,OILP=11,FINJ1=12,FINJ2=13,FINJ3=14,FINJ4=15,FINJ5=16,FINJ6=17,AINJ1=18,AINJ2=19,AINJ3=20,AINJ4=21,AINJ5=22,AINJ6=23,TACH=24,EST 1=36,EST 2=37,EST 3=38,EST 4=39,EST 5=40,EST 6=41,EST 7=42,EST 8=43  freq_mode=-1  min_freq=2  use_max_freq=off  max_freq=42949672.96  use_enable=off  use_brake=off  output_current=off  output_fault_status=off  use_child=off  use_vardec=on  nam='WASTEGATE'  read_level=1  write_level=1  group='System | I/O Pins | Outputs Config'
  wires:
  PWM Characterization/1 -> motohawk_pwm/1
  PWM Characterization/2 -> motohawk_pwm/2
  motohawk_fault_action/1 -> Logical Operator/1
  Product/1 -> PWM Characterization/1
  WASTEGATE/1 -> Product/1
  Logical Operator/1 -> Product/2

== system BaseEngineController_LS/Main Power Relay/Main Power Relay/Forced Shutdown Process ==
  ECUP State : Inport
  Logical Operator1 : Logic  Operator=NOT  OutDataTypeStr=boolean
  Logical Operator5 : Logic  Operator=NOT  OutDataTypeStr=boolean
  Post Shutdown two ticks before MPRD off : Subsystem  TreatAsAtomicUnit=on
  Processor Reboot : Subsystem  TreatAsAtomicUnit=on
  Relational Operator1 : RelationalOperator  OutDataTypeStr=boolean  ZeroCross=off  InputSameDT=on
  Save NV Vars one tick before MPRD off : Subsystem  TreatAsAtomicUnit=on
  Shutdown power on ECU565/563 : Subsystem  TreatAsAtomicUnit=on
  Time Since Enabled (With Input)1 : motohawk_control_primitives_lib/Time Since Enabled (With Input)1  SystemSampleTime=-1  nam='ForcedShutdown'  samp_time=-1  init=0  upperlim=16000
  Unit Delay6 : UnitDelay  SampleTime=-1
  Unit Delay7 : UnitDelay  SampleTime=-1
  Unit Delay8 : UnitDelay  SampleTime=-1
  motohawk_calibration1 : MotoHawk_lib/Calibration & Probing Blocks/motohawk_calibration  nam='ForcedShutDownTimerThresh'  val=12  storage=Calibration  show_more=on  name_source=Use Parameter  data_type=Inherit via back propagation  read_level=1  write_level=1  ovr_cals=on  view_as=Number  enum_struct={'Disabled', 'Enabled'}  vector_style=Wide Row  use_help_units=on  help='If ECUP is off for this time and application has not turned off, then force a shutdown routine.'  units='sec'  use_header_enum=off  row_header_enum={}  col_header_enum={}  use_min_max=on  min_val=0  max_val=1023  use_precision=off  precision=''  gain=1  offset=0  exp=1  use_mototune_group=on  mototune_group=motohawk_vardec_config_group(group)
  motohawk_probe1 : MotoHawk_lib/Calibration & Probing Blocks/motohawk_probe  nam='ForcedShutDownTimer'  show_more=on  name_source=Use Parameter  read_level=1  view_as=Number  enum_struct={'Disabled', 'Enabled'}  vector_style=Wide Row  use_help_units=off  help=''  units=''  use_header_enum=off  row_header_enum={}  col_header_enum={}  use_precision=off  precision=''  gain=1  offset=0  exp=1  use_mototune_group=on  mototune_group=group
  wires:
  Logical Operator1/1 -> Time Since Enabled (With Input)1/1
  ECUP State/1 -> Logical Operator1/1
  Unit Delay8/1 -> Processor Reboot/Trigger
  Logical Operator5/1 -> Post Shutdown two ticks before MPRD off/Trigger, Unit Delay6/1
  Unit Delay7/1 -> Shutdown power on ECU565/563/Trigger, Unit Delay8/1
  Unit Delay6/1 -> Unit Delay7/1, Save NV Vars one tick before MPRD off/Trigger
  Relational Operator1/1 -> Logical Operator5/1
  motohawk_calibration1/1 -> Relational Operator1/2
  Time Since Enabled (With Input)1/1 -> Relational Operator1/1, motohawk_probe1/1
